simulink model "metoda_splotowa"  (R2021b)
settings: Solver=FixedStepAuto  StartTime=0.0  StopTime=15  FixedStep=step_size  RelTol=1e-3
undefined symbols (not defined in the file or in its folder): A, B, C, D, K, phi, phi_1, phi_2, phi_3, step_size, T_iD
settings Model: NumberOfSteps=10  Creator=janja  LastModifiedBy=janja
settings SolverCC: ConcurrentTasks=on  PositivePriorityOrder=on
settings OptimizationCC: BlockReduction=off  DefaultParameterBehavior=Inlined  OptimizeBlockIOStorage=off  EnhancedBackFolding=on  PassReuseOutputArgsThreshold=0  InitFltsAndDblsToZero=on  OptimizeBlockOrder=speed  DifferentSizesBufferReuse=on
settings DebuggingCC: TasksWithSamePriorityMsg=none  ParameterTunabilityLossMsg=error  UnderSpecifiedDimensionMsg=error
settings HardwareCC: ProdLongLongMode=on  TargetLongLongMode=on
settings SFSimCC: SimTargetLang=C++
settings RTWCC: BuildConfiguration=Faster Runs
settings CodeAppCC: OperatorAnnotations=on

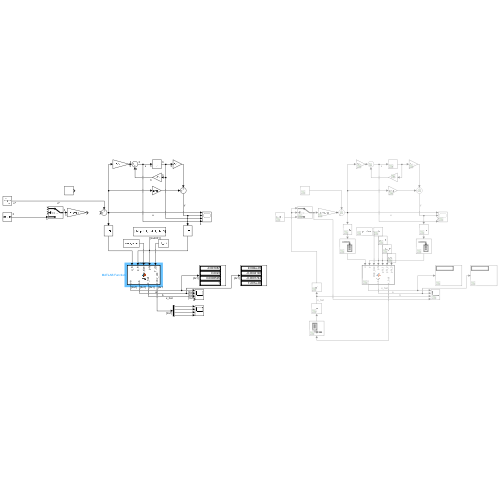
[thumbnail: Simulink's stored preview of the top-level diagram]
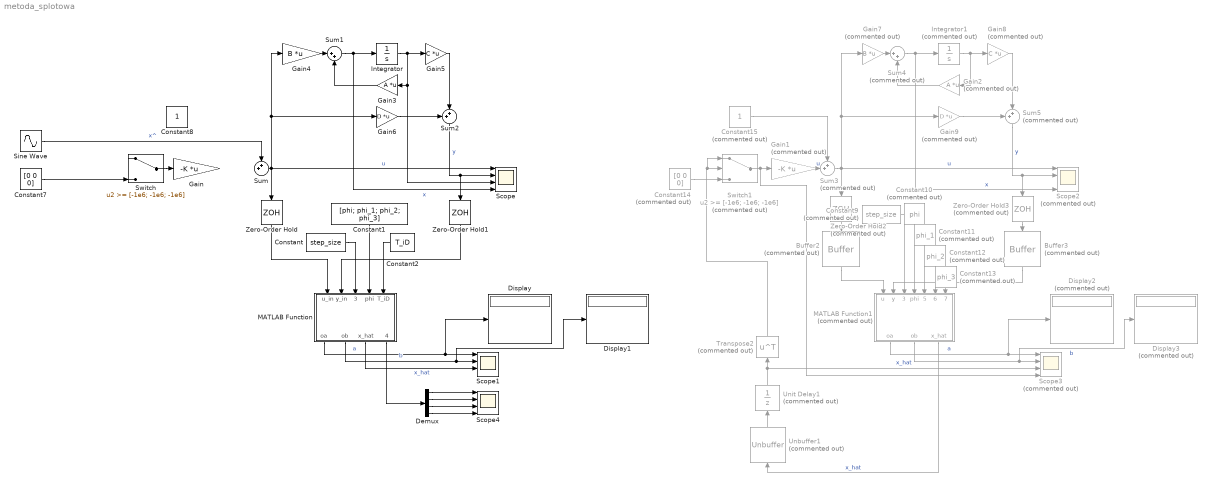
== system metoda_splotowa ==
  Buffer2 : Buffer  Commented=on  N=T_iD  V=T_iD-1  OutputFrames=off
  Buffer3 : Buffer  Commented=on  N=T_iD  V=T_iD-1  OutputFrames=off
  Constant : Constant  Value=step_size
  Constant1 : Constant  Value=[phi; phi_1; phi_2; phi_3]
  Constant10 : Constant  Commented=on  Value=phi
  Constant11 : Constant  Commented=on  Value=phi_1
  Constant12 : Constant  Commented=on  Value=phi_2
  Constant13 : Constant  Commented=on  Value=phi_3
  Constant14 : Constant  Commented=on  Value=[0 0 0]
  Constant15 : Constant  Commented=on
  Constant2 : Constant  Value=T_iD
  Constant7 : Constant  Value=[0 0 0]
  Constant8 : Constant
  Constant9 : Constant  Commented=on  Value=step_size
  Demux : Demux
  Display : Display
  Display1 : Display
  Display2 : Display  Commented=on
  Display3 : Display  Commented=on
  Gain : Gain  Gain=-K  Multiplication=Matrix(K*u) (u vector)
  Gain1 : Gain  Commented=on  Gain=-K  Multiplication=Matrix(K*u) (u vector)
  Gain2 : Gain  Commented=on  Gain=A  Multiplication=Matrix(K*u)
  Gain3 : Gain  Gain=A  Multiplication=Matrix(K*u)
  Gain4 : Gain  Gain=B  Multiplication=Matrix(K*u)
  Gain5 : Gain  Gain=C  Multiplication=Matrix(K*u)
  Gain6 : Gain  Gain=D  Multiplication=Matrix(K*u)
  Gain7 : Gain  Commented=on  Gain=B  Multiplication=Matrix(K*u)
  Gain8 : Gain  Commented=on  Gain=C  Multiplication=Matrix(K*u)
  Gain9 : Gain  Commented=on  Gain=D  Multiplication=Matrix(K*u)
  Integrator : Integrator  InitialCondition=[0 0 0]
  Integrator1 : Integrator  Commented=on  InitialCondition=[0 0 0]
  MATLAB Function : MATLAB Function  TreatAsAtomicUnit=on
  MATLAB Function1 : MATLAB Function  Commented=on  TreatAsAtomicUnit=on
  Scope : Scope  NumInputPorts=4
  Scope1 : Scope  NumInputPorts=4
  Scope2 : Scope  Commented=on  NumInputPorts=4
  Scope3 : Scope  Commented=on  NumInputPorts=4
  Scope4 : Scope  NumInputPorts=4
  Sine Wave : Sin  SampleTime=0
  Sum : Sum  Inputs=++|
  Sum1 : Sum  Inputs=|++
  Sum2 : Sum  Inputs=++|
  Sum3 : Sum  Commented=on  Inputs=++|
  Sum4 : Sum  Commented=on  Inputs=|++
  Sum5 : Sum  Commented=on  Inputs=++|
  Switch : Switch  Threshold=[-1e6; -1e6; -1e6]
  Switch1 : Switch  Commented=on  Threshold=[-1e6; -1e6; -1e6]
  Transpose2 : Math  Commented=on  Operator=transpose  OutputSignalType=real  SaturateOnIntegerOverflow=on
  Unbuffer1 : Unbuffer  Commented=on
  Unit Delay1 : UnitDelay  Commented=on  SampleTime=step_size  HasFrameUpgradeWarning=on
  Zero-Order Hold : ZeroOrderHold  SampleTime=step_size
  Zero-Order Hold1 : ZeroOrderHold  SampleTime=step_size
  Zero-Order Hold2 : ZeroOrderHold  Commented=on  SampleTime=step_size
  Zero-Order Hold3 : ZeroOrderHold  Commented=on  SampleTime=step_size
  wires:
  Integrator/1 -> Gain5/1, Scope/3, Gain3/1
  Gain4/1 -> Sum1/1
  Gain3/1 -> Sum1/2
  Sum1/1 -> Scope/4, Integrator/1  "x"
  Sum2/1 -> Zero-Order Hold1/1, Scope/2  "y"
  Gain5/1 -> Sum2/2
  Gain6/1 -> Sum2/1
  Zero-Order Hold/1 -> MATLAB Function/1(u_in)
  Zero-Order Hold1/1 -> MATLAB Function/2(y_in)
  Constant/1 -> MATLAB Function/3(step_size)
  MATLAB Function/2(ob) -> Display1/1, Scope1/2  "b"
  Constant1/1 -> MATLAB Function/4(phi)
  Switch/1 -> Gain/1
  MATLAB Function/1(oa) -> Display/1, Scope1/1  "a"
  Sum/1 -> Scope/1, Zero-Order Hold/1, Gain6/1, Gain4/1  "u"
  Constant7/1 -> Switch/3
  Constant10/1 -> MATLAB Function1/4(phi)
  Buffer2/1 -> MATLAB Function1/1(u)
  Unit Delay1/1 -> Scope3/3, Transpose2/1  "x_hat"
  Constant11/1 -> MATLAB Function1/5(phi_1)
  Switch1/1 -> Scope3/4, Gain1/1
  Zero-Order Hold3/1 -> Buffer3/1
  Gain9/1 -> Sum5/1
  Zero-Order Hold2/1 -> Buffer2/1
  Buffer3/1 -> MATLAB Function1/2(y)
  MATLAB Function1/2(ob) -> Display3/1, Scope3/2  "b"
  Sum5/1 -> Zero-Order Hold3/1, Scope2/2  "y"
  Sum4/1 -> Scope2/4, Integrator1/1  "x"
  Gain2/1 -> Sum4/2
  Constant9/1 -> MATLAB Function1/3(step_size)
  Gain1/1 -> Sum3/2  "u"
  MATLAB Function1/1(oa) -> Display2/1, Scope3/1  "a"
  Constant12/1 -> MATLAB Function1/6(phi_2)
  Transpose2/1 -> Switch1/1, Switch1/2
  Unbuffer1/1 -> Unit Delay1/1
  MATLAB Function1/3(x_hat) -> Unbuffer1/1  "x_hat"
  Constant14/1 -> Switch1/3
  Gain8/1 -> Sum5/2
  Sum3/1 -> Gain9/1, Gain7/1, Scope2/1, Zero-Order Hold2/1  "u"
  Gain7/1 -> Sum4/1
  Constant13/1 -> MATLAB Function1/7(phi_3)
  Constant15/1 -> Sum3/1
  Integrator1/1 -> Gain8/1, Gain2/1
  Sine Wave/1 -> Sum/1  "x^"
  MATLAB Function/3(x_hat) -> Scope1/3  "x_hat"
  Constant2/1 -> MATLAB Function/5(T_iD)
  MATLAB Function/4(conv_vec) -> Demux/1
  Demux/1 -> Scope4/1
  Demux/2 -> Scope4/2
  Demux/3 -> Scope4/3
  Demux/4 -> Scope4/4

== matlab function metoda_splotowa/MATLAB Function1 ==
  data: u input; oa output; y input; step_size input; ob output; phi input; phi_1 input; phi_2 input; phi_3 input; x_hat output
function [oa, ob, x_hat]= fcn(u, y, step_size, phi, phi_1, phi_2, phi_3)

%splot y*phi u*phi
h=length(phi);
T_iD=length(u);
y0=zeros(T_iD-h+1,1);
y1=zeros(T_iD-h+1,1);
y2=zeros(T_iD-h+1,1);
y3=zeros(T_iD-h+1,1);
u0=zeros(T_iD-h+1,1);
u1=zeros(T_iD-h+1,1);
u2=zeros(T_iD-h+1,1);
u3=zeros(T_iD-h+1,1);
t_=0:step_size:((2*h-2)*step_size);
for t_h=h:T_iD
    y0(t_h-h+1)=trapz(t_,conv(y(t_h-h+1:t_h),phi),1);
    y1(t_h-h+1)=trapz(t_,conv(y(t_h-h+1:t_h),phi_1),1);
    y2(t_h-h+1)=trapz(t_,conv(y(t_h-h+1:t_h),phi_2),1);
    y3(t_h-h+1)=trapz(t_,conv(y(t_h-h+1:t_h),phi_3),1);
    u0(t_h-h+1)=trapz(t_,conv(u(t_h-h+1:t_h),phi),1);
    u1(t_h-h+1)=trapz(t_,conv(u(t_h-h+1:t_h),phi_1),1);
    u2(t_h-h+1)=trapz(t_,conv(u(t_h-h+1:t_h),phi_2),1);
    u3(t_h-h+1)=trapz(t_,conv(u(t_h-h+1:t_h),phi_3),1);
end
% size=length(u0);
t=((h-1)*step_size):step_size:((T_iD-1)*step_size);
%integ(y*u dt) h->T => y(T)u(T) - y(h)u(h) - integ(y'integ(u) dt) h->T
% y0_prim=diff(y0)/step_size;
% y1_prim=diff(y1)/step_size;
% y2_prim=diff(y2)/step_size;
% y3_prim=diff(y3)/step_size;
% u0_prim=diff(u0)/step_size;
% u1_prim=diff(u1)/step_size;
% u2_prim=diff(u2)/step_size;
% u3_prim=diff(u3)/step_size;
% y0_integ=trapz(t,y0(1:end-1),1);
% y1_integ=trapz(t,y1(1:end-1),1);
% y2_integ=trapz(t,y2(1:end-1),1);
% y3_integ=trapz(t,y3(1:end-1),1);
% u0_integ=trapz(t,u0(1:end-1),1);
% u1_integ=trapz(t,u1(1:end-1),1);
% u2_integ=trapz(t,u2(1:end-1),1);
% u3_integ=trapz(t,u3(1:end-1),1);

% g11=y0(end)*y0(end) -y0(1)*y0(1) -trapz(t,y0_prim.*y0_integ,1);
% g12=y0(end)*y1(end) -y0(1)*y1(1) -trapz(t,y0_prim.*y1_integ,1);
% g13=y0(end)*y2(end) -y0(1)*y2(1) -trapz(t,y0_prim.*y2_integ,1);
% g14=y0(end)*y3(end) -y0(1)*y3(1) -trapz(t,y0_prim.*y3_integ,1);
% g15=y0(end)*u0(end) -y0(1)*u0(1) -trapz(t,y0_prim.*u0_integ,1);
% g16=y0(end)*u1(end) -y0(1)*u1(1) -trapz(t,y0_prim.*u1_integ,1);
% g17=y0(end)*u2(end) -y0(1)*u2(1) -trapz(t,y0_prim.*u2_integ,1);
% g18=y0(end)*u3(end) -y0(1)*u3(1) -trapz(t,y0_prim.*u3_integ,1);
% 
% g21=y1(end)*y0(end) -y1(1)*y0(1) -trapz(t,y1_prim.*y0_integ,1);
% g22=y1(end)*y1(end) -y1(1)*y1(1) -trapz(t,y1_prim.*y1_integ,1);
% g23=y1(end)*y2(end) -y1(1)*y2(1) -trapz(t,y1_prim.*y2_integ,1);
% g24=y1(end)*y3(end) -y1(1)*y3(1) -trapz(t,y1_prim.*y3_integ,1);
% g25=y1(end)*u0(end) -y1(1)*u0(1) -trapz(t,y1_prim.*u0_integ,1);
% g26=y1(end)*u1(end) -y1(1)*u1(1) -trapz(t,y1_prim.*u1_integ,1);
% g27=y1(end)*u2(end) -y1(1)*u2(1) -trapz(t,y1_prim.*u2_integ,1);
% g28=y1(end)*u3(end) -y1(1)*u3(1) -trapz(t,y1_prim.*u3_integ,1);
% 
% g31=y2(end)*y0(end) -y2(1)*y0(1) -trapz(t,y2_prim.*y0_integ,1);
% g32=y2(end)*y1(end) -y2(1)*y1(1) -trapz(t,y2_prim.*y1_integ,1);
% g33=y2(end)*y2(end) -y2(1)*y2(1) -trapz(t,y2_prim.*y2_integ,1);
% g34=y2(end)*y3(end) -y2(1)*y3(1) -trapz(t,y2_prim.*y3_integ,1);
% g35=y2(end)*u0(end) -y2(1)*u0(1) -trapz(t,y2_prim.*u0_integ,1);
% g36=y2(end)*u1(end) -y2(1)*u1(1) -trapz(t,y2_prim.*u1_integ,1);
% g37=y2(end)*u2(end) -y2(1)*u2(1) -trapz(t,y2_prim.*u2_integ,1);
% g38=y2(end)*u3(end) -y2(1)*u3(1) -trapz(t,y2_prim.*u3_integ,1);
% 
% g41=y3(end)*y0(end) -y3(1)*y0(1) -trapz(t,y3_prim.*y0_integ,1);
% g42=y3(end)*y1(end) -y3(1)*y1(1) -trapz(t,y3_prim.*y1_integ,1);
% g43=y3(end)*y2(end) -y3(1)*y2(1) -trapz(t,y3_prim.*y2_integ,1);
% g44=y3(end)*y3(end) -y3(1)*y3(1) -trapz(t,y3_prim.*y3_integ,1);
% g45=y3(end)*u0(end) -y3(1)*u0(1) -trapz(t,y3_prim.*u0_integ,1);
% g46=y3(end)*u1(end) -y3(1)*u1(1) -trapz(t,y3_prim.*u1_integ,1);
% g47=y3(end)*u2(end) -y3(1)*u2(1) -trapz(t,y3_prim.*u2_integ,1);
% g48=y3(end)*u3(end) -y3(1)*u3(1) -trapz(t,y3_prim.*u3_integ,1);
% 
% g51=u0(end)*y0(end) -u0(1)*y0(1) -trapz(t,u0_prim.*y0_integ,1);
% g52=u0(end)*y1(end) -u0(1)*y1(1) -trapz(t,u0_prim.*y1_integ,1);
% g53=u0(end)*y2(end) -u0(1)*y2(1) -trapz(t,u0_prim.*y2_integ,1);
% g54=u0(end)*y3(end) -u0(1)*y3(1) -trapz(t,u0_prim.*y3_integ,1);
% g55=u0(end)*u0(end) -u0(1)*u0(1) -trapz(t,u0_prim.*u0_integ,1);
% g56=u0(end)*u1(end) -u0(1)*u1(1) -trapz(t,u0_prim.*u1_integ,1);
% g57=u0(end)*u2(end) -u0(1)*u2(1) -trapz(t,u0_prim.*u2_integ,1);
% g58=u0(end)*u3(end) -u0(1)*u3(1) -trapz(t,u0_prim.*u3_integ,1);
% 
% g61=u1(end)*y0(end) -u1(1)*y0(1) -trapz(t,u1_prim.*y0_integ,1);
% g62=u1(end)*y1(end) -u1(1)*y1(1) -trapz(t,u1_prim.*y1_integ,1);
% g63=u1(end)*y2(end) -u1(1)*y2(1) -trapz(t,u1_prim.*y2_integ,1);
% g64=u1(end)*y3(end) -u1(1)*y3(1) -trapz(t,u1_prim.*y3_integ,1);
% g65=u1(end)*u0(end) -u1(1)*u0(1) -trapz(t,u1_prim.*u0_integ,1);
% g66=u1(end)*u1(end) -u1(1)*u1(1) -trapz(t,u1_prim.*u1_integ,1);
% g67=u1(end)*u2(end) -u1(1)*u2(1) -trapz(t,u1_prim.*u2_integ,1);
% g68=u1(end)*u3(end) -u1(1)*u3(1) -trapz(t,u1_prim.*u3_integ,1);
% 
% g71=u2(end)*y0(end) -u2(1)*y0(1) -trapz(t,u2_prim.*y0_integ,1);
% g72=u2(end)*y1(end) -u2(1)*y1(1) -trapz(t,u2_prim.*y1_integ,1);
% g73=u2(end)*y2(end) -u2(1)*y2(1) -trapz(t,u2_prim.*y2_integ,1);
% g74=u2(end)*y3(end) -u2(1)*y3(1) -trapz(t,u2_prim.*y3_integ,1);
% g75=u2(end)*u0(end) -u2(1)*u0(1) -trapz(t,u2_prim.*u0_integ,1);
% g76=u2(end)*u1(end) -u2(1)*u1(1) -trapz(t,u2_prim.*u1_integ,1);
% g77=u2(end)*u2(end) -u2(1)*u2(1) -trapz(t,u2_prim.*u2_integ,1);
% g78=u2(end)*u3(end) -u2(1)*u3(1) -trapz(t,u2_prim.*u3_integ,1);
% 
% g81=u3(end)*y0(end) -u3(1)*y0(1) -trapz(t,u3_prim.*y0_integ,1);
% g82=u3(end)*y1(end) -u3(1)*y1(1) -trapz(t,u3_prim.*y1_integ,1);
% g83=u3(end)*y2(end) -u3(1)*y2(1) -trapz(t,u3_prim.*y2_integ,1);
% g84=u3(end)*y3(end) -u3(1)*y3(1) -trapz(t,u3_prim.*y3_integ,1);
% g85=u3(end)*u0(end) -u3(1)*u0(1) -trapz(t,u3_prim.*u0_integ,1);
% g86=u3(end)*u1(end) -u3(1)*u1(1) -trapz(t,u3_prim.*u1_integ,1);
% g87=u3(end)*u2(end) -u3(1)*u2(1) -trapz(t,u3_prim.*u2_integ,1);
% g88=u3(end)*u3(end) -u3(1)*u3(1) -trapz(t,u3_prim.*u3_integ,1);

g11=trapz(t,y0.*y0,1);
g12=trapz(t,y0.*y1,1);
g13=trapz(t,y0.*y2,1);
g14=trapz(t,y0.*y3,1);
g15=trapz(t,y0.*u0,1);
g16=trapz(t,y0.*u1,1);
g17=trapz(t,y0.*u2,1);
g18=trapz(t,y0.*u3,1);

g21=trapz(t,y1.*y0,1);
g22=trapz(t,y1.*y1,1);
g23=trapz(t,y1.*y2,1);
g24=trapz(t,y1.*y3,1);
g25=trapz(t,y1.*u0,1);
g26=trapz(t,y1.*u1,1);
g27=trapz(t,y1.*u2,1);
g28=trapz(t,y1.*u3,1);

g31=trapz(t,y2.*y0,1);
g32=trapz(t,y2.*y1,1);
g33=trapz(t,y2.*y2,1);
g34=trapz(t,y2.*y3,1);
g35=trapz(t,y2.*u0,1);
g36=trapz(t,y2.*u1,1);
g37=trapz(t,y2.*u2,1);
g38=trapz(t,y2.*u3,1);

g41=trapz(t,y3.*y0,1);
g42=trapz(t,y3.*y1,1);
g43=trapz(t,y3.*y2,1);
g44=trapz(t,y3.*y3,1);
g45=trapz(t,y3.*u0,1);
g46=trapz(t,y3.*u1,1);
g47=trapz(t,y3.*u2,1);
g48=trapz(t,y3.*u3,1);

g51=trapz(t,u0.*y0,1);
g52=trapz(t,u0.*y1,1);
g53=trapz(t,u0.*y2,1);
g54=trapz(t,u0.*y3,1);
g55=trapz(t,u0.*u0,1);
g56=trapz(t,u0.*u1,1);
g57=trapz(t,u0.*u2,1);
g58=trapz(t,u0.*u3,1);

% g61=trapz(t,u1.*y0,1);
% g62=trapz(t,u1.*y1,1);
% g63=trapz(t,u1.*y2,1);
% g64=trapz(t,u1.*y3,1);
% g65=trapz(t,u1.*u0,1);
% g66=trapz(t,u1.*u1,1);
% g67=trapz(t,u1.*u2,1);
% g68=trapz(t,u1.*u3,1);
% 
% g71=trapz(t,u2.*y0,1);
% g72=trapz(t,u2.*y1,1);
% g73=trapz(t,u2.*y2,1);
% g74=trapz(t,u2.*y3,1);
% g75=trapz(t,u2.*u0,1);
% g76=trapz(t,u2.*u1,1);
% g77=trapz(t,u2.*u2,1);
% g78=trapz(t,u2.*u3,1);
% 
% g81=trapz(t,u3.*y0,1);
% g82=trapz(t,u3.*y1,1);
% g83=trapz(t,u3.*y2,1);
% g84=trapz(t,u3.*y3,1);
% g85=trapz(t,u3.*u0,1);
% g86=trapz(t,u3.*u1,1);
% g87=trapz(t,u3.*u2,1);
% g88=trapz(t,u3.*u3,1);

% G=[g11 g12 g13 g14 -g15 -g16 -g17 -g18;
%    g21 g22 g23 g24 -g25 -g26 -g27 -g28;
%    g31 g32 g33 g34 -g35 -g36 -g37 -g38;
%    g41 g42 g43 g44 -g45 -g46 -g47 -g48;
%    g51 g52 g53 g54 -g55 -g56 -g57 -g58;
%    g61 g62 g63 g64 -g65 -g66 -g67 -g68;
%    g71 g72 g73 g74 -g75 -g76 -g77 -g78;
%    g81 g82 g83 g84 -g85 -g86 -g87 -g88];

G=[g11 g12 g13 g14 -g15 ;
   g21 g22 g23 g24 -g25 ;
   g31 g32 g33 g34 -g35 ;
   g41 g42 g43 g44 -g45 ;
   g51 g52 g53 g54 -g55 ];

[V, D]=eig(G);
I=[0 0 0 0 0];
M=[1e6 1e6 1e6 1e6 1e6];
D=real(D);
V=real(V);
for j=1:length(D)
        for i=1:length(D)
            if i==j
                M(j)=D(i,j);
                I(j)=i;
            end
        end
end
ind=1;
for i=1:length(M)
    if abs(M(i))>1e-10 && min(M)==M(i)
        ind=i;
    end
end
%mogę identyfikować wszystkie a i b, później najwyżej się wyzerują
% oa=[V(4,1) V(3,1) V(2,1) V(1,1)];
% ob=[V(8,1) V(7,1) V(6,1) V(5,1)];

oa=[V(4,ind) V(3,ind) V(2,ind) V(1,ind)];
ob=[V(5,ind)];

H1=1/oa(1)*[oa(3) oa(2) oa(1) 0;
            oa(2) oa(1) 0 0;
            oa(1) 0 0 0];
% H2=1/oa(1)*[ob(3) ob(2) 0;
%             ob(2) 0 0;
%             0 0 0];
H2=1/oa(1)*[ob(1) 0 0;
            0 0 0;
            0 0 0];

% x_hat=real(transpose(H1*[y0';y1';y2';y3']-H2*[u0';u1';u2']));
x_hat=real(transpose(H1*[y0';y1';y2';y3']-H2*[u0';u1';u2']));

== matlab function metoda_splotowa/MATLAB Function ==
  data: u_in input; y_in input; step_size input; phi input; T_iD input; oa output; ob output; x_hat output; conv_vec output size=[4 1]
function [oa, ob, x_hat, conv_vec] = fcn(u_in, y_in, step_size, phi, T_iD)
persistent u_buff_local y_buff_local y0 y1 y2 y3 u0 u1 u2 u3
    oa=[0 0 0 0]';
    ob=[0 0 0 0]';
    x_hat=[0 0 0]';
    phi_0=phi(1,:)';
    phi_1=phi(2,:)';
    phi_2=phi(3,:)';
    phi_3=phi(4,:)';
    conv_vec=[0 0 0 0]';

%splot y*phi u*phi
h=length(phi_0);
if isempty(u_buff_local)
   u_buff_local=0;
   y_buff_local=0;
    y0=0;
    y1=0;
    y2=0;
    y3=0;
    u0=0;
    u1=0;
    u2=0;
    u3=0;
else
    u_buff_local=[u_buff_local; u_in];
    y_buff_local=[y_buff_local; y_in];
    y0 = [y0; 0];
    y1 = [y1; 0];
    y2 = [y2; 0];
    y3 = [y3; 0];
    u0 = [u0; 0];
    u1 = [u1; 0];
    u2 = [u2; 0];
    u3 = [u3; 0];
    len_u=length(u_buff_local);
    len_y=length(y_buff_local);
    if len_u>=h && len_y>=h
        if len_u>T_iD && len_y>T_iD
            u_buff_local=u_buff_local(end-T_iD+1:end);
            y_buff_local=y_buff_local(end-T_iD+1:end);
            y0 = y0(end-T_iD+1:end);
            y1 = y1(end-T_iD+1:end);
            y2 = y2(end-T_iD+1:end);
            y3 = y3(end-T_iD+1:end);
            u0 = u0(end-T_iD+1:end);
            u1 = u1(end-T_iD+1:end);
            u2 = u2(end-T_iD+1:end);
            u3 = u3(end-T_iD+1:end);
        end
        u=u_buff_local;
        y=y_buff_local;
%         y0=zeros(length(y_buff_local)-h+1,1);
%         y1=zeros(length(y_buff_local)-h+1,1);
%         y2=zeros(length(y_buff_local)-h+1,1);
%         y3=zeros(length(y_buff_local)-h+1,1);
%         u0=zeros(length(u_buff_local)-h+1,1);
%         u1=zeros(length(u_buff_local)-h+1,1);
%         u2=zeros(length(u_buff_local)-h+1,1);
%         u3=zeros(length(u_buff_local)-h+1,1);
        t_=0:step_size:((h-1)*step_size);
%         for t_h=h:length(y)
%             y0(t_h-h+1)=trapz(t_,(y(t_h-h+1:t_h).*flipud(phi_0)),1);
%             y1(t_h-h+1)=trapz(t_,(y(t_h-h+1:t_h).*flipud(phi_1)),1);
%             y2(t_h-h+1)=trapz(t_,(y(t_h-h+1:t_h).*flipud(phi_2)),1);
%             y3(t_h-h+1)=trapz(t_,(y(t_h-h+1:t_h).*flipud(phi_3)),1);
%             u0(t_h-h+1)=trapz(t_,(u(t_h-h+1:t_h).*flipud(phi_0)),1);
%             u1(t_h-h+1)=trapz(t_,(u(t_h-h+1:t_h).*flipud(phi_1)),1);
%             u2(t_h-h+1)=trapz(t_,(u(t_h-h+1:t_h).*flipud(phi_2)),1);
%             u3(t_h-h+1)=trapz(t_,(u(t_h-h+1:t_h).*flipud(phi_3)),1);
%         end

%%persistent variables
        y0(end)=trapz(t_,(y(end-h+1:end).*flipud(phi_0)),1);
        y1(end)=trapz(t_,(y(end-h+1:end).*flipud(phi_1)),1);
        y2(end)=trapz(t_,(y(end-h+1:end).*flipud(phi_2)),1);
        y3(end)=trapz(t_,(y(end-h+1:end).*flipud(phi_3)),1);
        u0(end)=trapz(t_,(u(end-h+1:end).*flipud(phi_0)),1);
        u1(end)=trapz(t_,(u(end-h+1:end).*flipud(phi_1)),1);
        u2(end)=trapz(t_,(u(end-h+1:end).*flipud(phi_2)),1);
        u3(end)=trapz(t_,(u(end-h+1:end).*flipud(phi_3)),1);

%         for t_h=h:length(y)
%             y0(t_h-h+1)=trapz(t_,conv(y(t_h-h+1:t_h),phi_0),1);
%             y1(t_h-h+1)=trapz(t_,conv(y(t_h-h+1:t_h),phi_1),1);
%             y2(t_h-h+1)=trapz(t_,conv(y(t_h-h+1:t_h),phi_2),1);
%             y3(t_h-h+1)=trapz(t_,conv(y(t_h-h+1:t_h),phi_3),1);
%             u0(t_h-h+1)=trapz(t_,conv(u(t_h-h+1:t_h),phi_0),1);
%             u1(t_h-h+1)=trapz(t_,conv(u(t_h-h+1:t_h),phi_1),1);
%             u2(t_h-h+1)=trapz(t_,conv(u(t_h-h+1:t_h),phi_2),1);
%             u3(t_h-h+1)=trapz(t_,conv(u(t_h-h+1:t_h),phi_3),1);
%         end

%         y0=conv(y(end-h+1:end),phi_0);
%         y1=conv(y(end-h+1:end),phi_1);
%         y2=conv(y(end-h+1:end),phi_2);
%         y3=conv(y(end-h+1:end),phi_3);
%         u0=conv(u(end-h+1:end),phi_0);
%         u1=conv(u(end-h+1:end),phi_1);
%         u2=conv(u(end-h+1:end),phi_2);
%         u3=conv(u(end-h+1:end),phi_3);
        conv_vec=[y0(end) y1(end) y2(end) y3(end)]';
        % size=length(u0);
        t=0:step_size:((length(y0)-1)*step_size);
        %integ(y*u dt) h->T => y(T)u(T) - y(h)u(h) - integ(y'integ(u) dt) h->T
        % y0_prim=diff(y0)/step_size;
        % y1_prim=diff(y1)/step_size;
        % y2_prim=diff(y2)/step_size;
        % y3_prim=diff(y3)/step_size;
        % u0_prim=diff(u0)/step_size;
        % u1_prim=diff(u1)/step_size;
        % u2_prim=diff(u2)/step_size;
        % u3_prim=diff(u3)/step_size;
        % y0_integ=trapz(t,y0(1:end-1),1);
        % y1_integ=trapz(t,y1(1:end-1),1);
        % y2_integ=trapz(t,y2(1:end-1),1);
        % y3_integ=trapz(t,y3(1:end-1),1);
        % u0_integ=trapz(t,u0(1:end-1),1);
        % u1_integ=trapz(t,u1(1:end-1),1);
        % u2_integ=trapz(t,u2(1:end-1),1);
        % u3_integ=trapz(t,u3(1:end-1),1);
        
        % g11=y0(end)*y0(end) -y0(1)*y0(1) -trapz(t,y0_prim.*y0_integ,1);
        % g12=y0(end)*y1(end) -y0(1)*y1(1) -trapz(t,y0_prim.*y1_integ,1);
        % g13=y0(end)*y2(end) -y0(1)*y2(1) -trapz(t,y0_prim.*y2_integ,1);
        % g14=y0(end)*y3(end) -y0(1)*y3(1) -trapz(t,y0_prim.*y3_integ,1);
        % g15=y0(end)*u0(end) -y0(1)*u0(1) -trapz(t,y0_prim.*u0_integ,1);
        % g16=y0(end)*u1(end) -y0(1)*u1(1) -trapz(t,y0_prim.*u1_integ,1);
        % g17=y0(end)*u2(end) -y0(1)*u2(1) -trapz(t,y0_prim.*u2_integ,1);
        % g18=y0(end)*u3(end) -y0(1)*u3(1) -trapz(t,y0_prim.*u3_integ,1);
        % 
        % g21=y1(end)*y0(end) -y1(1)*y0(1) -trapz(t,y1_prim.*y0_integ,1);
        % g22=y1(end)*y1(end) -y1(1)*y1(1) -trapz(t,y1_prim.*y1_integ,1);
        % g23=y1(end)*y2(end) -y1(1)*y2(1) -trapz(t,y1_prim.*y2_integ,1);
        % g24=y1(end)*y3(end) -y1(1)*y3(1) -trapz(t,y1_prim.*y3_integ,1);
        % g25=y1(end)*u0(end) -y1(1)*u0(1) -trapz(t,y1_prim.*u0_integ,1);
        % g26=y1(end)*u1(end) -y1(1)*u1(1) -trapz(t,y1_prim.*u1_integ,1);
        % g27=y1(end)*u2(end) -y1(1)*u2(1) -trapz(t,y1_prim.*u2_integ,1);
        % g28=y1(end)*u3(end) -y1(1)*u3(1) -trapz(t,y1_prim.*u3_integ,1);
        % 
        % g31=y2(end)*y0(end) -y2(1)*y0(1) -trapz(t,y2_prim.*y0_integ,1);
        % g32=y2(end)*y1(end) -y2(1)*y1(1) -trapz(t,y2_prim.*y1_integ,1);
        % g33=y2(end)*y2(end) -y2(1)*y2(1) -trapz(t,y2_prim.*y2_integ,1);
        % g34=y2(end)*y3(end) -y2(1)*y3(1) -trapz(t,y2_prim.*y3_integ,1);
        % g35=y2(end)*u0(end) -y2(1)*u0(1) -trapz(t,y2_prim.*u0_integ,1);
        % g36=y2(end)*u1(end) -y2(1)*u1(1) -trapz(t,y2_prim.*u1_integ,1);
        % g37=y2(end)*u2(end) -y2(1)*u2(1) -trapz(t,y2_prim.*u2_integ,1);
        % g38=y2(end)*u3(end) -y2(1)*u3(1) -trapz(t,y2_prim.*u3_integ,1);
        % 
        % g41=y3(end)*y0(end) -y3(1)*y0(1) -trapz(t,y3_prim.*y0_integ,1);
        % g42=y3(end)*y1(end) -y3(1)*y1(1) -trapz(t,y3_prim.*y1_integ,1);
        % g43=y3(end)*y2(end) -y3(1)*y2(1) -trapz(t,y3_prim.*y2_integ,1);
        % g44=y3(end)*y3(end) -y3(1)*y3(1) -trapz(t,y3_prim.*y3_integ,1);
        % g45=y3(end)*u0(end) -y3(1)*u0(1) -trapz(t,y3_prim.*u0_integ,1);
        % g46=y3(end)*u1(end) -y3(1)*u1(1) -trapz(t,y3_prim.*u1_integ,1);
        % g47=y3(end)*u2(end) -y3(1)*u2(1) -trapz(t,y3_prim.*u2_integ,1);
        % g48=y3(end)*u3(end) -y3(1)*u3(1) -trapz(t,y3_prim.*u3_integ,1);
        % 
        % g51=u0(end)*y0(end) -u0(1)*y0(1) -trapz(t,u0_prim.*y0_integ,1);
        % g52=u0(end)*y1(end) -u0(1)*y1(1) -trapz(t,u0_prim.*y1_integ,1);
        % g53=u0(end)*y2(end) -u0(1)*y2(1) -trapz(t,u0_prim.*y2_integ,1);
        % g54=u0(end)*y3(end) -u0(1)*y3(1) -trapz(t,u0_prim.*y3_integ,1);
        % g55=u0(end)*u0(end) -u0(1)*u0(1) -trapz(t,u0_prim.*u0_integ,1);
        % g56=u0(end)*u1(end) -u0(1)*u1(1) -trapz(t,u0_prim.*u1_integ,1);
        % g57=u0(end)*u2(end) -u0(1)*u2(1) -trapz(t,u0_prim.*u2_integ,1);
        % g58=u0(end)*u3(end) -u0(1)*u3(1) -trapz(t,u0_prim.*u3_integ,1);
        % 
        % g61=u1(end)*y0(end) -u1(1)*y0(1) -trapz(t,u1_prim.*y0_integ,1);
        % g62=u1(end)*y1(end) -u1(1)*y1(1) -trapz(t,u1_prim.*y1_integ,1);
        % g63=u1(end)*y2(end) -u1(1)*y2(1) -trapz(t,u1_prim.*y2_integ,1);
        % g64=u1(end)*y3(end) -u1(1)*y3(1) -trapz(t,u1_prim.*y3_integ,1);
        % g65=u1(end)*u0(end) -u1(1)*u0(1) -trapz(t,u1_prim.*u0_integ,1);
        % g66=u1(end)*u1(end) -u1(1)*u1(1) -trapz(t,u1_prim.*u1_integ,1);
        % g67=u1(end)*u2(end) -u1(1)*u2(1) -trapz(t,u1_prim.*u2_integ,1);
        % g68=u1(end)*u3(end) -u1(1)*u3(1) -trapz(t,u1_prim.*u3_integ,1);
        % 
        % g71=u2(end)*y0(end) -u2(1)*y0(1) -trapz(t,u2_prim.*y0_integ,1);
        % g72=u2(end)*y1(end) -u2(1)*y1(1) -trapz(t,u2_prim.*y1_integ,1);
        % g73=u2(end)*y2(end) -u2(1)*y2(1) -trapz(t,u2_prim.*y2_integ,1);
        % g74=u2(end)*y3(end) -u2(1)*y3(1) -trapz(t,u2_prim.*y3_integ,1);
        % g75=u2(end)*u0(end) -u2(1)*u0(1) -trapz(t,u2_prim.*u0_integ,1);
        % g76=u2(end)*u1(end) -u2(1)*u1(1) -trapz(t,u2_prim.*u1_integ,1);
        % g77=u2(end)*u2(end) -u2(1)*u2(1) -trapz(t,u2_prim.*u2_integ,1);
        % g78=u2(end)*u3(end) -u2(1)*u3(1) -trapz(t,u2_prim.*u3_integ,1);
        % 
        % g81=u3(end)*y0(end) -u3(1)*y0(1) -trapz(t,u3_prim.*y0_integ,1);
        % g82=u3(end)*y1(end) -u3(1)*y1(1) -trapz(t,u3_prim.*y1_integ,1);
        % g83=u3(end)*y2(end) -u3(1)*y2(1) -trapz(t,u3_prim.*y2_integ,1);
        % g84=u3(end)*y3(end) -u3(1)*y3(1) -trapz(t,u3_prim.*y3_integ,1);
        % g85=u3(end)*u0(end) -u3(1)*u0(1) -trapz(t,u3_prim.*u0_integ,1);
        % g86=u3(end)*u1(end) -u3(1)*u1(1) -trapz(t,u3_prim.*u1_integ,1);
        % g87=u3(end)*u2(end) -u3(1)*u2(1) -trapz(t,u3_prim.*u2_integ,1);
        % g88=u3(end)*u3(end) -u3(1)*u3(1) -trapz(t,u3_prim.*u3_integ,1);
        
        g11=trapz(t,y0.*y0,1);
        g12=trapz(t,y0.*y1,1);
        g13=trapz(t,y0.*y2,1);
        g14=trapz(t,y0.*y3,1);
        g15=trapz(t,y0.*u0,1);
        g16=trapz(t,y0.*u1,1);
        g17=trapz(t,y0.*u2,1);
        g18=trapz(t,y0.*u3,1);
        
%         g21=trapz(t,y1.*y0,1);
        g22=trapz(t,y1.*y1,1);
        g23=trapz(t,y1.*y2,1);
        g24=trapz(t,y1.*y3,1);
        g25=trapz(t,y1.*u0,1);
        g26=trapz(t,y1.*u1,1);
        g27=trapz(t,y1.*u2,1);
        g28=trapz(t,y1.*u3,1);
        
%         g31=trapz(t,y2.*y0,1);
%         g32=trapz(t,y2.*y1,1);
        g33=trapz(t,y2.*y2,1);
        g34=trapz(t,y2.*y3,1);
        g35=trapz(t,y2.*u0,1);
        g36=trapz(t,y2.*u1,1);
        g37=trapz(t,y2.*u2,1);
        g38=trapz(t,y2.*u3,1);
        
%         g41=trapz(t,y3.*y0,1);
%         g42=trapz(t,y3.*y1,1);
%         g43=trapz(t,y3.*y2,1);
        g44=trapz(t,y3.*y3,1);
        g45=trapz(t,y3.*u0,1);
        g46=trapz(t,y3.*u1,1);
        g47=trapz(t,y3.*u2,1);
        g48=trapz(t,y3.*u3,1);
        
%         g51=trapz(t,u0.*y0,1);
%         g52=trapz(t,u0.*y1,1);
%         g53=trapz(t,u0.*y2,1);
%         g54=trapz(t,u0.*y3,1);
        g55=trapz(t,u0.*u0,1);
        g56=trapz(t,u0.*u1,1);
        g57=trapz(t,u0.*u2,1);
        g58=trapz(t,u0.*u3,1);
        
        % g61=trapz(t,u1.*y0,1);
        % g62=trapz(t,u1.*y1,1);
        % g63=trapz(t,u1.*y2,1);
        % g64=trapz(t,u1.*y3,1);
        % g65=trapz(t,u1.*u0,1);
        g66=trapz(t,u1.*u1,1);
        g67=trapz(t,u1.*u2,1);
        g68=trapz(t,u1.*u3,1);
        % 
        % g71=trapz(t,u2.*y0,1);
        % g72=trapz(t,u2.*y1,1);
        % g73=trapz(t,u2.*y2,1);
        % g74=trapz(t,u2.*y3,1);
        % g75=trapz(t,u2.*u0,1);
        % g76=trapz(t,u2.*u1,1);
        g77=trapz(t,u2.*u2,1);
        g78=trapz(t,u2.*u3,1);
        % 
        % g81=trapz(t,u3.*y0,1);
        % g82=trapz(t,u3.*y1,1);
        % g83=trapz(t,u3.*y2,1);
        % g84=trapz(t,u3.*y3,1);
        % g85=trapz(t,u3.*u0,1);
        % g86=trapz(t,u3.*u1,1);
        % g87=trapz(t,u3.*u2,1);
        g88=trapz(t,u3.*u3,1);
        
        G=[g11 g12 g13 g14 -g15 -g16 -g17 -g18;
           g12 g22 g23 g24 -g25 -g26 -g27 -g28;
           g13 g23 g33 g34 -g35 -g36 -g37 -g38;
           g14 g24 g34 g44 -g45 -g46 -g47 -g48;
           -g15 -g25 -g35 -g45 g55 g56 g57 g58;
           -g16 -g26 -g36 -g46 g56 g66 g67 g68;
           -g17 -g27 -g37 -g47 g57 g67 g77 g78;
           -g18 -g28 -g38 -g48 g58 g68 g78 g88];
        
%         G=[g11 g12 g13 g14 -g15 ;
%            g12 g22 g23 g24 -g25 ;
%            g13 g23 g33 g34 -g35 ;
%            g14 g24 g34 g44 -g45 ;
%            -g15 -g25 -g35 -g45 g55 ];
        
        [V, D]=eig(G);
        I=[0 0 0 0 0 0 0 0];
        M=[1e6 1e6 1e6 1e6 1e6 1e6 1e6 1e6];
        D=real(D);
        V=real(V);
        for j=1:length(D)
            for i=1:length(D)
                if i==j
                    M(j)=D(i,j);
                    I(j)=i;
                end
            end
        end
        ind=1;
        temp_min=1e6;
        for i=1:length(M)
            if  M(i)<temp_min %&& abs(M(i))>1e-10 
                ind=i;
                temp_min=M(ind);
            end
        end
        %mogę identyfikować wszystkie a i b, później najwyżej się wyzerują
        % oa=[V(4,1) V(3,1) V(2,1) V(1,1)];
        % ob=[V(8,1) V(7,1) V(6,1) V(5,1)];
%         V=abs(V);
        oa=[V(4,ind) V(3,ind) V(2,ind) V(1,ind)]';
        ob=[V(8,ind) V(7,ind) V(6,ind) V(5,ind)]';
        
        H1=1/oa(1)*[oa(3) oa(2) oa(1) 0;
                    oa(2) oa(1) 0 0;
                    oa(1) 0 0 0];
%         H2=1/oa(1)*[ob(3) ob(2) 0;
%                     ob(2) 0 0;
%                     0 0 0];
        H2=1/oa(1)*[ob(1) 0 0;
                    0 0 0;
                    0 0 0];
        
        x_temp=real(transpose(H1*[y0';y1';y2';y3']-H2*[u0';u1';u2']));
        x_hat=x_temp(end,:)';
    end
end
